simulink model "AHRS_voter"  (R2019a)
settings: Solver=FixedStepDiscrete  StartTime=0.0  StopTime=10.0  FixedStep=0.01  RelTol=1e-3  EnableMultiTasking=on
libraries: simulink x1
Description:
  | This model implements a voting algorithm for three AHRS.  Depending on the number of valid AHRS, the system will provide a mid value, an average value or a single value.
settings Model: DataDictionary=HeliSystemDD.sldd  Creator=bpotter  LastModifiedBy=bpotter
settings DataIOCC: LimitDataPoints=on  SaveFormat=Array  ReturnWorkspaceOutputs=off
settings OptimizationCC: BlockReduction=off  ConditionallyExecuteInputs=off  DefaultParameterBehavior=Inlined  UseDivisionForNetSlopeComputation=on  InitFltsAndDblsToZero=on  EfficientFloat2IntCast=on  EfficientMapNaN2IntZero=off  LifeSpan=inf  MaxStackSize=inf
settings DebuggingCC: SignalInfNanChecking=error  SignalRangeChecking=error  ReadBeforeWriteMsg=EnableAllAsError  WriteAfterWriteMsg=EnableAllAsError  WriteAfterReadMsg=EnableAllAsError  AlgebraicLoopMsg=error  ArtificialAlgebraicLoopMsg=error  SaveWithDisabledLinksMsg=error  SaveWithParameterizedLinksMsg=error  BlockPriorityViolationMsg=error  SolverPrmCheckMsg=error  InheritedTsInSrcMsg=error  SingleTaskRateTransMsg=error  TasksWithSamePriorityMsg=error  SigSpecEnsureSampleTimeMsg=error  CheckMatrixSingularityMsg=error  IntegerOverflowMsg=error  ParameterUnderflowMsg=error  ParameterPrecisionLossMsg=error  ParameterTunabilityLossMsg=error  UnderSpecifiedDataTypeMsg=error  UnnecessaryDatatypeConvMsg=warning  VectorMatrixConversionMsg=error  SignalLabelMismatchMsg=error  UnconnectedInputMsg=error  UnconnectedOutputMsg=error  UnconnectedLineMsg=error  SFcnCompatibilityMsg=error  UniqueDataStoreMsg=error  BusObjectLabelMismatch=error  RootOutportRequireBusObject=error  AssertControl=DisableAll  AllowSymbolicDim=off  ModelReferenceIOMsg=error  ModelReferenceIOMismatchMessage=error  UnknownTsInhSupMsg=error  ModelReferenceDataLoggingMessage=error  StateNameClashWarn=warning  PregeneratedLibrarySubsystemCodeDiagnostic=none  StrictBusMsg=ErrorOnBusTreatedAsVector  NonBusSignalsTreatedAsBus=error  SFInvalidInputDataAccessInChartInitDiag=error  SFTransitionOutsideNaturalParentDiag=error  SFUnreachableExecutionPathDiag=error  SFUndirectedBroadcastEventsDiag=error  SFTransitionActionBeforeConditionDiag=error  SFExecutionAtInitializationDiag=none  IntegerSaturationMsg=error  ArithmeticOperatorsInVariantConditions=warning
settings HardwareCC: ProdBitPerPointer=32  ProdBitPerSizeT=32  ProdBitPerPtrDiffT=32  ProdWordSize=32  ProdHWDeviceType=Intel->x86-32 (Windows32)  TargetIntDivRoundTo=Zero
settings ModelReferenceCC: ModelReferenceNumInstancesAllowed=Single  PropagateSignalLabelsOutOfModel=off
settings SFSimCC: SimUseLocalCustomCode=off  CompileTimeRecursionLimit=0  EnableRuntimeRecursion=off  MATLABDynamicMemAlloc=off
settings RTWCC: SystemTargetFile=ert.tlc  TemplateMakefile=ert_default_tmf  GenerateReport=on  RTWUseLocalCustomCode=off  IncludeHyperlinkInReport=on  LaunchReport=on  PortableWordSizes=on  GenerateTraceInfo=on  GenerateTraceReport=on  GenerateTraceReportSl=on  GenerateTraceReportSf=on  GenerateTraceReportEml=on
settings CodeAppCC: ForceParamTrailComments=on  IgnoreCustomStorageClasses=off  MATLABFcnDesc=on  MangleLength=4  StateflowObjectComments=on  ReqsInCode=on
settings ERTTargetCC: TargetLangStandard=C99 (ISO)  UtilityFuncGeneration=Shared location  MultiwordLength=2048  GenerateSampleERTMain=on  IncludeMdlTerminateFcn=off  SuppressErrorStatus=on  SupportAbsoluteTime=off  SupportNonFinite=off  ParenthesesLevel=Maximum  CastingMode=Standards  GenerateSharedConstants=off  ERTCustomFileTemplate=example_file_process.tlc  ERTFilePackagingFormat=Compact  PreserveExpressionOrder=on  PreserveIfCondition=on  ConvertIfToSwitch=off  SuppressUnreachableDefaultCases=off  EnableSignedLeftShifts=off  EnableSignedRightShifts=off
settings ConfigComp: CovEnable=on  RecordCoverage=on  CovMetricSettings=dcmtrzoibe  CovHTMLOptions=-sRT=1 -sVT=0 -aTS=1 -bRG=1 -bTC=1 -hTR=1 -nFC=0 -scm=1 -bcm=1 -xEv=0  CovSaveCumulativeToWorkspaceVar=on  CovCumulativeVarName=AHRScovCumData  CovCumulativeReport=on  CovModelRefEnable=on  CovExternalEMLEnable=off  CovSFcnEnable=off  PSVerificationMode=BugFinder  PSResultDir=\BugFinder_results  PSModelRefVerifDepth=All  PSAutoStubLUT=off  DVMakeOutputFilesUnique=off  DVModelCoverageObjectives=MCDC  DVTestSuiteOptimization=IndividualObjectives  DVIgnoreCovSatisfied=on  DVCoverageDataFile=simulation_results\AHRS_voter_cov.cvt  DVIncludeRelationalBoundary=on  DVSaveDataFile=off  DVSaveReport=on  DVReportPDFFormat=on  DVRebuildModelRepresentation=Always

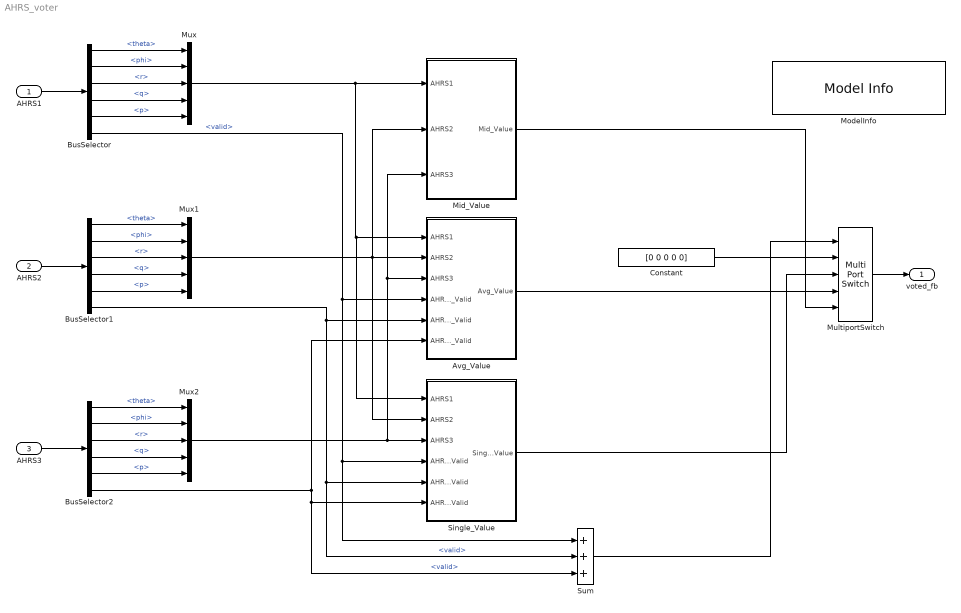
== system AHRS_voter ==
  AHRS1 : Inport  RequirementInfo={} %GIDa_0e6f3d6a_507d_4b38_9a17_e8cee3262a0c  OutDataTypeStr=Bus: AHRS_Bus  PortDimensions=1  SampleTime=0.01  BusOutputAsStruct=on
  AHRS2 : Inport  RequirementInfo={} %GIDa_4f9d425b_1c2a_4e63_860c_37d1f8e2e588  Port=2  OutDataTypeStr=Bus: AHRS_Bus  PortDimensions=1  SampleTime=0.01  BusOutputAsStruct=on
  AHRS3 : Inport  RequirementInfo={} %GIDa_c75126fd_43b0_47dc_a702_928eb5a31267  Port=3  OutDataTypeStr=Bus: AHRS_Bus  PortDimensions=1  SampleTime=0.01  BusOutputAsStruct=on
  Avg_Value : Subsystem  RequirementInfo={} %GIDa_f27afd25_99ab_4174_a01a_4860294926e6  TreatAsAtomicUnit=on  RTWFcnName=Avg_Value
      settings: RTWSystemCode=Inline  RTWFcnNameOpts=User specified
  BusSelector : BusSelector  OutputSignals=theta,phi,r,q,p,valid
  BusSelector1 : BusSelector  OutputSignals=theta,phi,r,q,p,valid
  BusSelector2 : BusSelector  OutputSignals=theta,phi,r,q,p,valid
  Constant : Constant  Value=[0 0 0 0 0]
  Mid_Value : Subsystem  RequirementInfo={} %GIDa_08f08dd7_7cca_494c_808e_b4d628beaa7c  TreatAsAtomicUnit=on  RTWFcnName=Mid_Value
      settings: RTWSystemCode=Inline  RTWFcnNameOpts=User specified
  ModelInfo : simulink/Model-Wide Utilities/Model Info  Frame=on  DisplayStringWithTags=|  HorizontalTextAlignment=Center  LeftAlignmentValue=0.5
      | Model Name: %<ModelName>
      | Model Version: %<ModelVersion>
      | Last Modified: %<LastModificationDate>
      | 
      | Copyright 2016 The MathWorks, Inc.
  MultiportSwitch : MultiPortSwitch  RequirementInfo={} %GIDa_519e60fb_1ec7_4a47_a883_2bbbc7544923  DataPortOrder=Zero-based contiguous  Inputs=4  DiagnosticForDefault=None  zeroidx=on
  Mux : Mux  Inputs=5
  Mux1 : Mux  Inputs=5
  Mux2 : Mux  Inputs=5
  Single_Value : Subsystem  RequirementInfo={} %GIDa_b324ce75_7724_488b_996f_30db6bdf9d28  TreatAsAtomicUnit=on  RTWFcnName=Single_Value
      settings: RTWSystemCode=Inline  RTWFcnNameOpts=User specified
  Sum : Sum  RequirementInfo={} %GIDa_9e079f55_0fbd_4328_aeec_4d524e6f1f82  Inputs=+++  OutDataTypeStr=uint32
  voted_fb : Outport  RequirementInfo={} %GIDa_54a7513f_600a_4d69_b144_1552dbc20ce0
  wires:
  MultiportSwitch/1 -> voted_fb/1
  Sum/1 -> MultiportSwitch/1
  Mid_Value/1(Mid_Value) -> MultiportSwitch/5
  Avg_Value/1(Avg_Value) -> MultiportSwitch/4
  Single_Value/1(Single_Value) -> MultiportSwitch/3
  Constant/1 -> MultiportSwitch/2
  AHRS1/1 -> BusSelector/1
  BusSelector/6 -> Single_Value/4(AHRS1_Valid), Sum/1, Avg_Value/4(AHRS1_Valid)  "<valid>"
  BusSelector/1 -> Mux/1  "<theta>"
  BusSelector/2 -> Mux/2  "<phi>"
  BusSelector/3 -> Mux/3  "<r>"
  BusSelector/4 -> Mux/4  "<q>"
  BusSelector/5 -> Mux/5  "<p>"
  Mux/1 -> Single_Value/1(AHRS1), Avg_Value/1(AHRS1), Mid_Value/1(AHRS1)
  BusSelector1/5 -> Mux1/5  "<p>"
  BusSelector1/4 -> Mux1/4  "<q>"
  BusSelector1/3 -> Mux1/3  "<r>"
  BusSelector1/2 -> Mux1/2  "<phi>"
  BusSelector1/1 -> Mux1/1  "<theta>"
  AHRS2/1 -> BusSelector1/1
  Mux1/1 -> Single_Value/2(AHRS2), Mid_Value/2(AHRS2), Avg_Value/2(AHRS2)
  BusSelector1/6 -> Avg_Value/5(AHRS2_Valid), Sum/2, Single_Value/5(AHRS2_Valid)  "<valid>"
  Mux2/1 -> Mid_Value/3(AHRS3), Avg_Value/3(AHRS3), Single_Value/3(AHRS3)
  AHRS3/1 -> BusSelector2/1
  BusSelector2/1 -> Mux2/1  "<theta>"
  BusSelector2/2 -> Mux2/2  "<phi>"
  BusSelector2/3 -> Mux2/3  "<r>"
  BusSelector2/4 -> Mux2/4  "<q>"
  BusSelector2/5 -> Mux2/5  "<p>"
  BusSelector2/6 -> Single_Value/6(AHRS3_Valid), Sum/3, Avg_Value/6(AHRS3_Valid)  "<valid>"

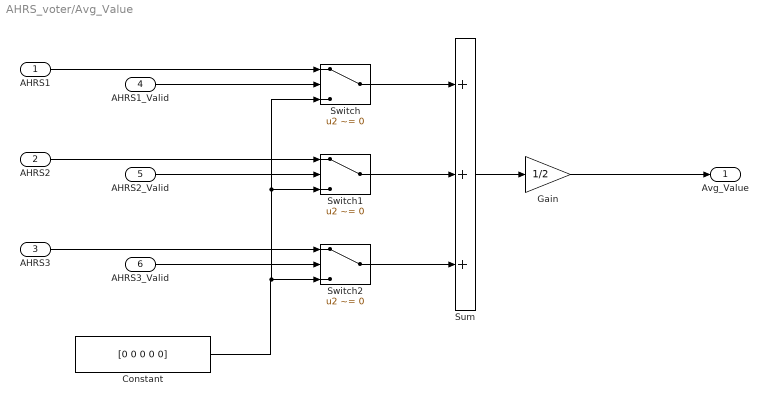
== system AHRS_voter/Avg_Value ==
  AHRS1 : Inport  RequirementInfo={} %GIDa_1d3a7457_8bba_4b66_94a4_9b91d2894b41
  AHRS2 : Inport  RequirementInfo={} %GIDa_ad2f1df6_f413_49fd_a7fc_2ffba44399b5  Port=2
  AHRS3 : Inport  RequirementInfo={} %GIDa_d87833b2_9372_47b9_8ab4_d90850f3ceab  Port=3
  AHRS1_Valid : Inport  RequirementInfo={} %GIDa_d720385a_f274_4a8e_b8c8_c8af340df28d  Port=4  OutDataTypeStr=boolean  PortDimensions=1
  AHRS2_Valid : Inport  RequirementInfo={} %GIDa_a5c2b44c_83ae_4397_97c3_240b44d0f31e  Port=5  OutDataTypeStr=boolean  PortDimensions=1
  AHRS3_Valid : Inport  RequirementInfo={} %GIDa_ce68107c_0c52_40f4_96e8_5bc14e1666a3  Port=6  OutDataTypeStr=boolean  PortDimensions=1
  Constant : Constant  RequirementInfo={} %GIDa_1baaca7a_567b_421d_9bf3_d97f8a899f88  Value=[0 0 0 0 0]
  Gain : Gain  RequirementInfo={} %GIDa_744273b4_a4b5_45b9_a127_68b0bf2cfe21  Gain=1/2
  Sum : Sum  RequirementInfo={} %GIDa_72402a66_151b_4b06_b0a5_cb869a9f2fb3  Inputs=+++
  Switch : Switch  RequirementInfo={} %GIDa_dd846285_d555_4115_9230_f91bafdc094a  Criteria=u2 ~= 0
  Switch1 : Switch  RequirementInfo={} %GIDa_45c43aef_2e9e_49f2_b096_4a10b5458d02  Criteria=u2 ~= 0
  Switch2 : Switch  RequirementInfo={} %GIDa_5b010bfc_353f_4e8f_8bb6_ad9ebd83dc36  Criteria=u2 ~= 0
  Avg_Value : Outport  RequirementInfo={} %GIDa_610fdf2b_6797_497d_8da2_e35043b8fbe6
  wires:
  Gain/1 -> Avg_Value/1
  Sum/1 -> Gain/1
  AHRS1_Valid/1 -> Switch/2
  AHRS1/1 -> Switch/1
  Switch/1 -> Sum/1
  Switch1/1 -> Sum/2
  Switch2/1 -> Sum/3
  AHRS2_Valid/1 -> Switch1/2
  AHRS3_Valid/1 -> Switch2/2
  AHRS2/1 -> Switch1/1
  AHRS3/1 -> Switch2/1
  Constant/1 -> Switch/3, Switch1/3, Switch2/3

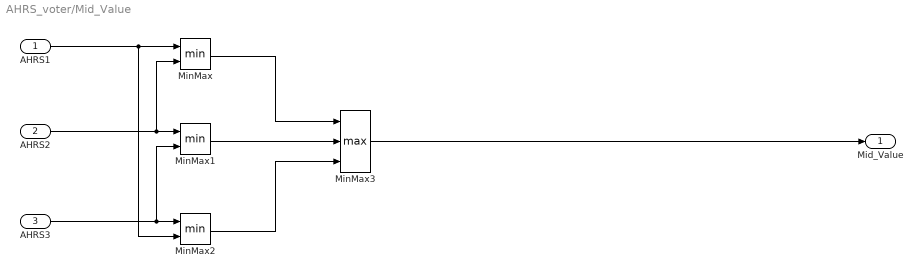
== system AHRS_voter/Mid_Value ==
  AHRS1 : Inport  RequirementInfo={} %GIDa_90684716_0f12_41a5_ba06_7045a06f2f9d
  AHRS2 : Inport  RequirementInfo={} %GIDa_3738c67e_b0fd_4e71_aadc_e147e6eff95b  Port=2
  AHRS3 : Inport  RequirementInfo={} %GIDa_f02eb8bb_cdb6_4039_9857_c1cf4d006570  Port=3
  MinMax : MinMax  RequirementInfo={} %GIDa_04162a78_ca1a_4bca_a8e0_7af3205f29d7  Inputs=2
  MinMax1 : MinMax  RequirementInfo={} %GIDa_b7200490_7e5a_4849_b6d3_458b16996efd  Inputs=2
  MinMax2 : MinMax  RequirementInfo={} %GIDa_ca34bc0d_15d3_492b_a57c_74313d597f5d  Inputs=2
  MinMax3 : MinMax  RequirementInfo={} %GIDa_39cfa399_63b3_488b_a528_95912ba9519b  Function=max  Inputs=3
  Mid_Value : Outport  RequirementInfo={} %GIDa_4a45428f_3218_44d8_acb8_483625c59e19
  wires:
  AHRS1/1 -> MinMax2/2, MinMax/1
  AHRS3/1 -> MinMax1/2, MinMax2/1
  AHRS2/1 -> MinMax/2, MinMax1/1
  MinMax1/1 -> MinMax3/2
  MinMax/1 -> MinMax3/1
  MinMax2/1 -> MinMax3/3
  MinMax3/1 -> Mid_Value/1

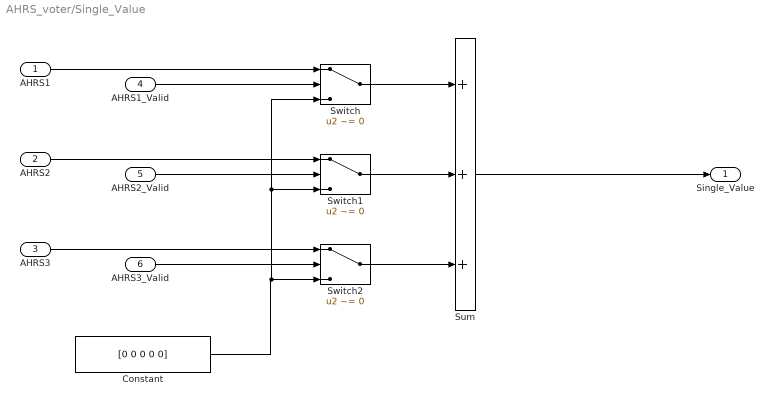
== system AHRS_voter/Single_Value ==
  AHRS1 : Inport  RequirementInfo={} %GIDa_8c8cb7e3_10e4_4703_b756_6019f10f2a68
  AHRS2 : Inport  RequirementInfo={} %GIDa_64a3edb7_5e0d_458d_ac73_c7e9c514ccb6  Port=2
  AHRS3 : Inport  RequirementInfo={} %GIDa_a2b6e9a1_8c1d_4b16_a103_423b7668c7fb  Port=3
  AHRS1_Valid : Inport  RequirementInfo={} %GIDa_ba6b2ee9_52f9_40b9_b5c3_1702be58441f  Port=4  OutDataTypeStr=boolean  PortDimensions=1
  AHRS2_Valid : Inport  RequirementInfo={} %GIDa_de85ca1f_f90b_4100_bdaa_c92379d7ac93  Port=5  OutDataTypeStr=boolean  PortDimensions=1
  AHRS3_Valid : Inport  RequirementInfo={} %GIDa_5f64fbdb_c064_4f1a_aca7_89de324ee3a6  Port=6  OutDataTypeStr=boolean  PortDimensions=1
  Constant : Constant  RequirementInfo={} %GIDa_ed9b2c54_364e_49c0_a0bc_1892a31a6930  Value=[0 0 0 0 0]
  Sum : Sum  RequirementInfo={} %GIDa_04460614_0acd_4063_a654_a3d0a585fb23  Inputs=+++
  Switch : Switch  RequirementInfo={} %GIDa_e1e98aa7_da83_4611_b1ce_9e54a1eeac9d  Criteria=u2 ~= 0
  Switch1 : Switch  RequirementInfo={} %GIDa_47388979_ee51_454e_b4ca_04a21024ae04  Criteria=u2 ~= 0
  Switch2 : Switch  RequirementInfo={} %GIDa_2f5b568c_d619_4b1e_9da4_e347d6673694  Criteria=u2 ~= 0
  Single_Value : Outport  RequirementInfo={} %GIDa_91ee2a03_2d0f_4193_92cb_d92f10ae47b8
  wires:
  Constant/1 -> Switch2/3, Switch1/3, Switch/3
  AHRS3/1 -> Switch2/1
  AHRS2/1 -> Switch1/1
  AHRS3_Valid/1 -> Switch2/2
  AHRS2_Valid/1 -> Switch1/2
  Switch2/1 -> Sum/3
  Switch1/1 -> Sum/2
  Switch/1 -> Sum/1
  AHRS1/1 -> Switch/1
  AHRS1_Valid/1 -> Switch/2
  Sum/1 -> Single_Value/1
